simulink model "Colorspace_Conversion_fixed_start"  (R2025a)
settings: Solver=VariableStepAuto  StartTime=0.0  StopTime=10  RelTol=1e-3  EnableMultiTasking=on
undefined symbols (not defined in the file): gray
libraries: hlsBasic x23, dspvision x1
settings Model: Creator=ukumar  LastModifiedBy=robg
settings SolverCC: AlgebraicLoopSolver=TrustRegion
settings DataIOCC: ReturnWorkspaceOutputs=off
settings OptimizationCC: LifeSpan=inf
settings DebuggingCC: InheritedTsInSrcMsg=none  UnconnectedInputMsg=warning  UnconnectedOutputMsg=warning  UnconnectedLineMsg=warning  SFUnexpectedBacktrackingDiag=warning  SFNoUnconditionalDefaultTransitionDiag=warning  ArithmeticOperatorsInVariantConditions=warning
settings ModelReferenceCC: EnableRefExpFcnMdlSchedulingChecks=on
settings SFSimCC: SimUseLocalCustomCode=off  CustomCodeUndefinedFunction=UseInterfaceOnly
settings RTWCC: RTWUseLocalCustomCode=off  GPUComputeCapability=3.5
settings CodeAppCC: StateflowObjectComments=on
settings GRTTargetCC: TargetLangStandard=C89/C90 (ANSI)
settings ConfigComp: CovMetricSettings=dw  CovSaveCumulativeToWorkspaceVar=on  CovSaveSingleToWorkspaceVar=on  CovExternalEMLEnable=off

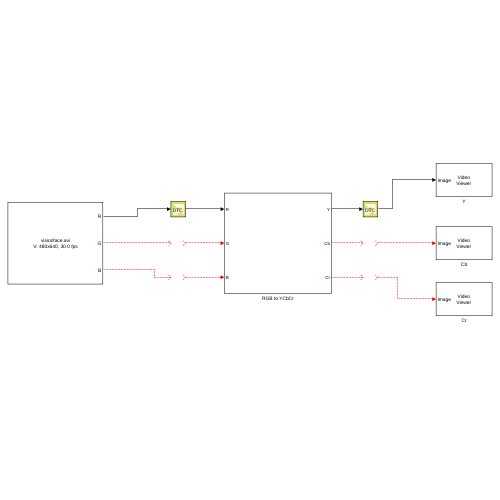
[thumbnail: Simulink's stored preview of the top-level diagram]
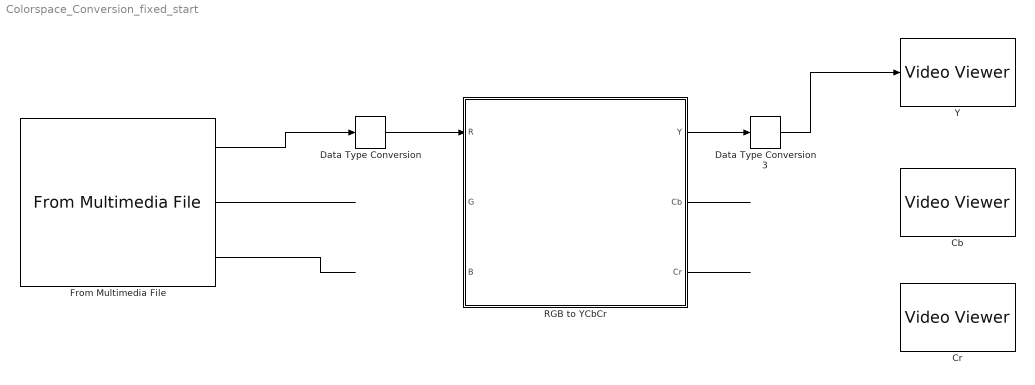
== system Colorspace_Conversion_fixed_start ==
  "Cb " : VideoViewer  colormapValue=gray(256)  FigPos=[23.4 519.6 487.2 356]
  "Cr " : VideoViewer  colormapValue=gray(256)  FigPos=[534.6 513.2 460.8 352]
  Data Type Conversion : hlsBasic/Data Type Conversion  OutDataType=double  TypeExp=''  Signedness=Signed  WordLength=16  FractionalLength=10  RoundingMode=Truncation to minus infinity  OverflowMode=Wrap around
  Data Type Conversion3 : hlsBasic/Data Type Conversion  OutDataType=double  TypeExp=''  Signedness=Signed  WordLength=16  FractionalLength=10  RoundingMode=Truncation to minus infinity  OverflowMode=Wrap around
  From Multimedia File : dspvision/From Multimedia File  inputFilename=visionface.avi  readRange=[1 Inf]  loop=on  numPlays=inf  outputStreams=Video only  videoDataType=single  audioDataType=int16  inheritSampleTime=on  userDefinedSampleTime=1/30  noAudioOutput=off  isIntensityVideo=off  fourcc=RGB  colorVideoFormat=Separate color signals  outputEOF=off  dataOrg=Column-major  audioFrameSize=1024  computeAudioFrameSize=off  outSamplingMode=Sample based
  RGB to YCbCr : Subsystem
  Y : VideoViewer  colormapValue=gray(256)  FigPos=[1016.2 530.8 471.2 368.8]
  wires:
  From Multimedia File/2 -> ?
  From Multimedia File/3 -> ?
  RGB to YCbCr/1(Y) -> Data Type Conversion3/1
  RGB to YCbCr/2(Cb) -> ?
  RGB to YCbCr/3(Cr) -> ?
  From Multimedia File/1 -> Data Type Conversion/1
  Data Type Conversion/1 -> RGB to YCbCr/1(R)
  ? -> RGB to YCbCr/2(G)
  ? -> RGB to YCbCr/3(B)
  Data Type Conversion3/1 -> Y/1
  ? -> "Cb "/1
  ? -> "Cr "/1

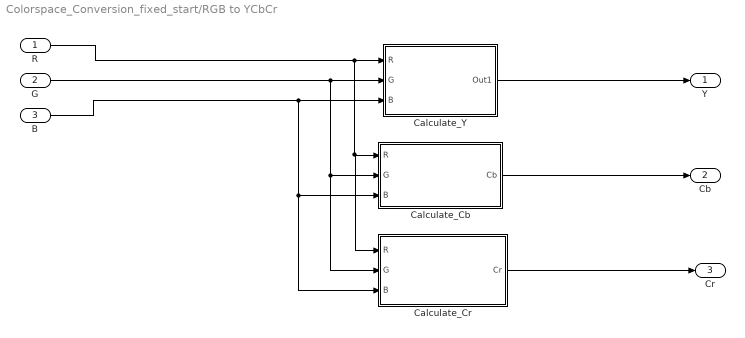
== system Colorspace_Conversion_fixed_start/RGB to YCbCr ==
  R : Inport
  G : Inport  Port=2
  B : Inport  Port=3
  "Calculate_Cb " : Subsystem
  Calculate_Cr : Subsystem
  "Calculate_Y " : Subsystem
  Y : Outport
  Cb : Outport  Port=2
  Cr : Outport  Port=3
  wires:
  "Calculate_Y "/1(Out1) -> Y/1
  "Calculate_Cb "/1("Cb ") -> Cb/1
  Calculate_Cr/1(Cr) -> Cr/1
  R/1 -> Calculate_Cr/1("R "), "Calculate_Cb "/1("R "), "Calculate_Y "/1("R ")
  G/1 -> Calculate_Cr/2("G "), "Calculate_Cb "/2("G "), "Calculate_Y "/2("G ")
  B/1 -> Calculate_Cr/3(B), "Calculate_Cb "/3(B), "Calculate_Y "/3("B ")

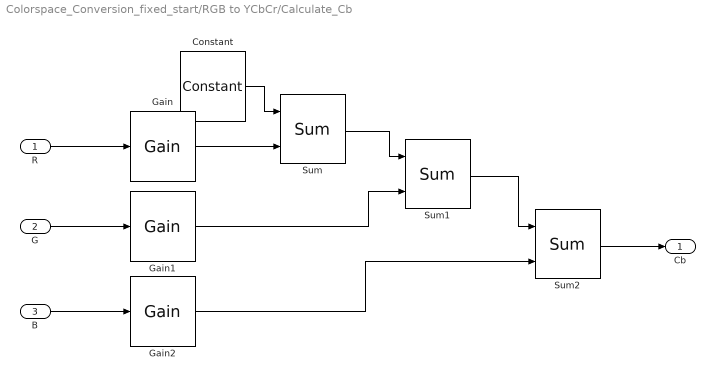
== system Colorspace_Conversion_fixed_start/RGB to YCbCr/Calculate_Cb  ==
  "R " : Inport
  "G " : Inport  Port=2
  B : Inport  Port=3
  Constant : hlsBasic/Constant  Description=Performs multiplication  Value=128/255  VectorParams1D=off  SampleTime=-1  OutDataType=single  TypeExp=''  Signedness=Signed  WordLength=16  FractionalLength=0  RoundingMode=Truncation to minus infinity  OverflowMode=Wrap around
  Gain : hlsBasic/Gain  Description=Performs multiplication  Gain=-37.945/256  OutDataType=single  TypeExp=''  Signedness=Signed  WordLength=5  FractionalLength=4  RoundingMode=Truncation to minus infinity  OverflowMode=Wrap around  OutputTypeAsInput=off
  Gain1 : hlsBasic/Gain  Description=Performs multiplication  Gain=-74.494/256  OutDataType=single  TypeExp=''  Signedness=Signed  WordLength=5  FractionalLength=4  RoundingMode=Truncation to minus infinity  OverflowMode=Wrap around  OutputTypeAsInput=off
  Gain2 : hlsBasic/Gain  Description=Performs multiplication  Gain=112.439/256  OutDataType=single  TypeExp=''  Signedness=Signed  WordLength=5  FractionalLength=4  RoundingMode=Truncation to minus infinity  OverflowMode=Wrap around  OutputTypeAsInput=off
  Sum : hlsBasic/Sum
  Sum1 : hlsBasic/Sum
  Sum2 : hlsBasic/Sum
  "Cb " : Outport
  wires:
  Sum2/1 -> "Cb "/1
  "R "/1 -> Gain/1
  "G "/1 -> Gain1/1
  B/1 -> Gain2/1
  Constant/1 -> Sum/1
  Gain/1 -> Sum/2
  Sum/1 -> Sum1/1
  Gain1/1 -> Sum1/2
  Sum1/1 -> Sum2/1
  Gain2/1 -> Sum2/2

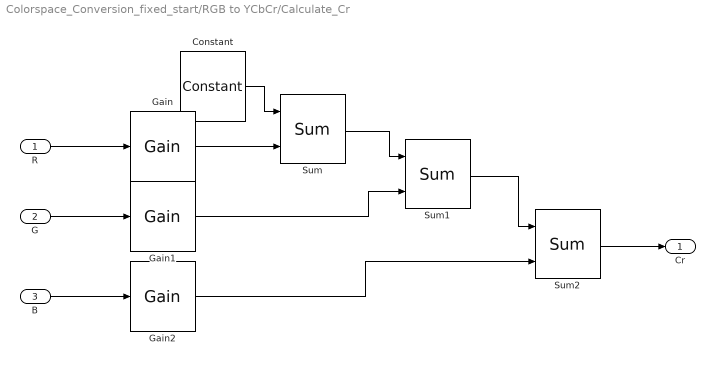
== system Colorspace_Conversion_fixed_start/RGB to YCbCr/Calculate_Cr ==
  "R " : Inport
  "G " : Inport  Port=2
  B : Inport  Port=3
  Constant : hlsBasic/Constant  Description=Performs multiplication  Value=128/255  VectorParams1D=off  SampleTime=-1  OutDataType=single  TypeExp=''  Signedness=Signed  WordLength=16  FractionalLength=0  RoundingMode=Truncation to minus infinity  OverflowMode=Wrap around
  Gain : hlsBasic/Gain  Description=Performs multiplication  Gain=112.439/256  OutDataType=single  TypeExp=''  Signedness=Signed  WordLength=5  FractionalLength=4  RoundingMode=Truncation to minus infinity  OverflowMode=Wrap around  OutputTypeAsInput=off
  Gain1 : hlsBasic/Gain  Description=Performs multiplication  Gain=-94.154/256  OutDataType=single  TypeExp=''  Signedness=Signed  WordLength=5  FractionalLength=4  RoundingMode=Truncation to minus infinity  OverflowMode=Wrap around  OutputTypeAsInput=off
  Gain2 : hlsBasic/Gain  Description=Performs multiplication  Gain=-18.285/256  OutDataType=single  TypeExp=''  Signedness=Signed  WordLength=5  FractionalLength=4  RoundingMode=Truncation to minus infinity  OverflowMode=Wrap around  OutputTypeAsInput=off
  Sum : hlsBasic/Sum
  Sum1 : hlsBasic/Sum
  Sum2 : hlsBasic/Sum
  Cr : Outport
  wires:
  Gain2/1 -> Sum2/2
  Sum1/1 -> Sum2/1
  Gain1/1 -> Sum1/2
  Sum/1 -> Sum1/1
  Gain/1 -> Sum/2
  Constant/1 -> Sum/1
  B/1 -> Gain2/1
  "G "/1 -> Gain1/1
  "R "/1 -> Gain/1
  Sum2/1 -> Cr/1

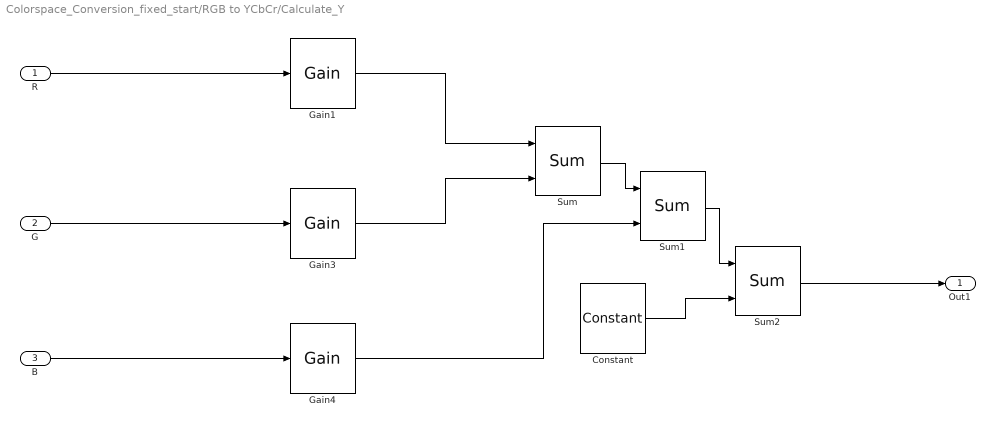
== system Colorspace_Conversion_fixed_start/RGB to YCbCr/Calculate_Y  ==
  "R " : Inport
  "G " : Inport  Port=2
  "B " : Inport  Port=3
  Constant : hlsBasic/Constant  Description=Performs multiplication  Value=16/255  VectorParams1D=off  SampleTime=-1  OutDataType=single  TypeExp=''  Signedness=Signed  WordLength=16  FractionalLength=0  RoundingMode=Truncation to minus infinity  OverflowMode=Wrap around
  Gain1 : hlsBasic/Gain  Description=Performs multiplication  Gain=65.738/256  OutDataType=single  TypeExp=''  Signedness=Signed  WordLength=5  FractionalLength=4  RoundingMode=Truncation to minus infinity  OverflowMode=Wrap around  OutputTypeAsInput=off
  Gain3 : hlsBasic/Gain  Description=Performs multiplication  Gain=129.057/256  OutDataType=single  TypeExp=''  Signedness=Signed  WordLength=5  FractionalLength=4  RoundingMode=Truncation to minus infinity  OverflowMode=Wrap around  OutputTypeAsInput=off
  Gain4 : hlsBasic/Gain  Description=Performs multiplication  Gain=25.064/256  OutDataType=single  TypeExp=''  Signedness=Signed  WordLength=5  FractionalLength=4  RoundingMode=Truncation to minus infinity  OverflowMode=Wrap around  OutputTypeAsInput=off
  Sum : hlsBasic/Sum
  Sum1 : hlsBasic/Sum
  Sum2 : hlsBasic/Sum
  Out1 : Outport
  wires:
  Sum/1 -> Sum1/1
  "R "/1 -> Gain1/1
  "B "/1 -> Gain4/1
  "G "/1 -> Gain3/1
  Gain1/1 -> Sum/1
  Gain3/1 -> Sum/2
  Gain4/1 -> Sum1/2
  Sum1/1 -> Sum2/1
  Constant/1 -> Sum2/2
  Sum2/1 -> Out1/1
